simulink library "three_phase_dab_modulator"  (R2025b)
settings: Solver=VariableStepAuto  StartTime=0.0  StopTime=10.0  RelTol=1e-3
undefined symbols (not defined in the file): tc
libraries: SV_pattern_generator_with_global_TRGO x2
settings Model: Creator=dbagn  LastModifiedBy=dbagn

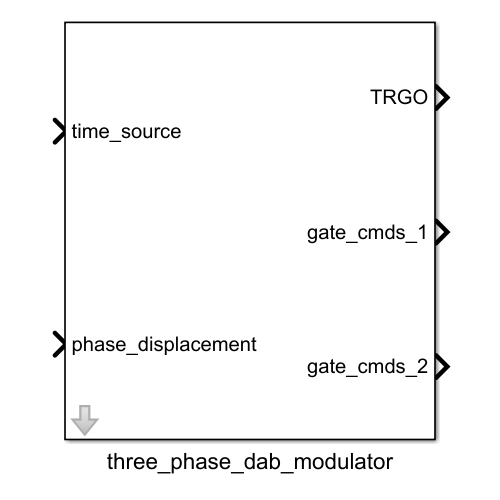
[thumbnail: Simulink's stored preview of the top-level diagram]
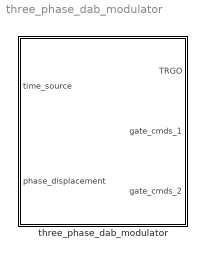
== system three_phase_dab_modulator ==
  three_phase_dab_modulator : Subsystem  mask{fpwm=2400, dead_time=0, tc=tc}
      mask prompts: fpwm "fpwm (Hz)"; dead_time "dead_time (s)"; tc "sampling time (s)"

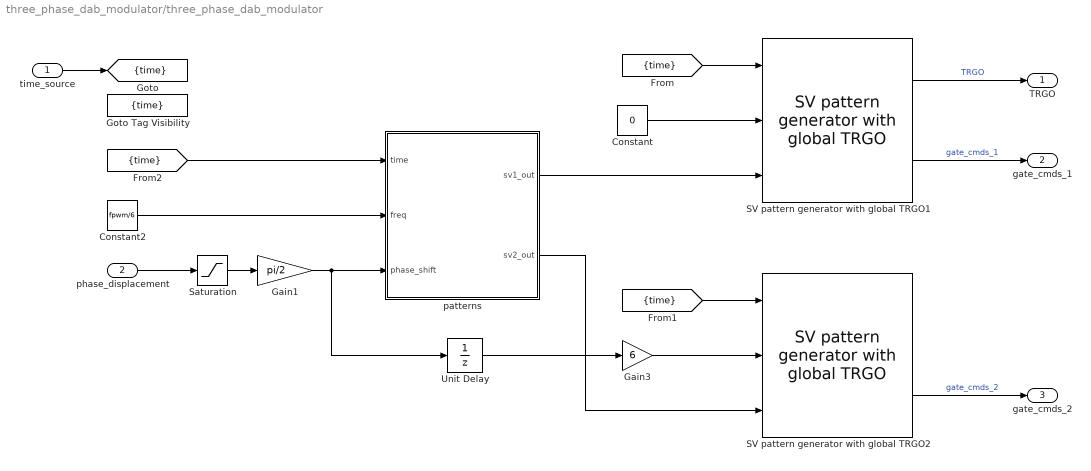
== system three_phase_dab_modulator/three_phase_dab_modulator ==
  time_source : Inport
  phase_displacement : Inport  Port=2
  Constant : Constant  Value=0
  Constant2 : Constant  Value=fpwm/6
  Gain1 : Gain  Gain=pi/2
  Gain3 : Gain  Gain=6
  Goto Tag Visibility : GotoTagVisibility  GotoTag=time
  SV pattern generator with global TRGO1 : SV_pattern_generator_with_global_TRGO/SV pattern generator with global TRGO  f=fpwm  m_up=0.98  m_low=0.02  dead_time=dead_time  pos_cmd_gate=15  neg_cmd_gate=-10  tc=tc
  SV pattern generator with global TRGO2 : SV_pattern_generator_with_global_TRGO/SV pattern generator with global TRGO  f=fpwm  m_up=0.98  m_low=0.02  dead_time=dead_time  pos_cmd_gate=15  neg_cmd_gate=-10  tc=tc
  Saturation : Saturate  UpperLimit=1  LowerLimit=-1
  Unit Delay : UnitDelay  SampleTime=tc  HasFrameUpgradeWarning=on
  patterns : Subsystem
  TRGO : Outport
  gate_cmds_1 : Outport  Port=2
  gate_cmds_2 : Outport  Port=3
  tag scope: time=scoped
  wires:
  SV pattern generator with global TRGO1/2 -> gate_cmds_1/1  "gate_cmds_1"
  Gain3/1 -> SV pattern generator with global TRGO2/2
  Constant/1 -> SV pattern generator with global TRGO1/2
  Constant2/1 -> patterns/2(freq)
  patterns/2(sv2_out) -> SV pattern generator with global TRGO2/3
  patterns/1(sv1_out) -> SV pattern generator with global TRGO1/3
  SV pattern generator with global TRGO1/1 -> TRGO/1  "TRGO"
  phase_displacement/1 -> Saturation/1
  SV pattern generator with global TRGO2/2 -> gate_cmds_2/1  "gate_cmds_2"
  time_source/1 -> [time]
  [time] -> SV pattern generator with global TRGO1/1
  [time] -> SV pattern generator with global TRGO2/1
  [time] -> patterns/1(time)
  Unit Delay/1 -> Gain3/1
  Gain1/1 -> Unit Delay/1, patterns/3(phase_shift)
  Saturation/1 -> Gain1/1

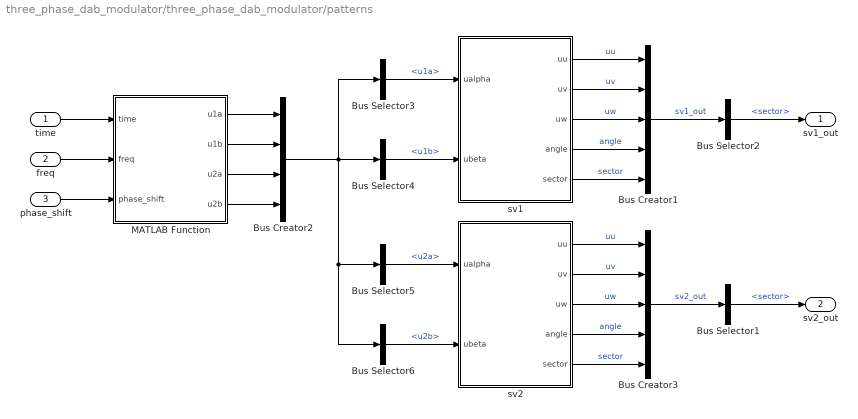
== system three_phase_dab_modulator/three_phase_dab_modulator/patterns ==
  time : Inport
  freq : Inport  Port=2
  phase_shift : Inport  Port=3
  Bus Creator1 : BusCreator  Inputs=5
  Bus Creator2 : BusCreator  Inputs=4
  Bus Creator3 : BusCreator  Inputs=5
  Bus Selector1 : BusSelector  OutputSignals=sector
  Bus Selector2 : BusSelector  OutputSignals=sector
  Bus Selector3 : BusSelector  OutputSignals=u1a
  Bus Selector4 : BusSelector  OutputSignals=u1b
  Bus Selector5 : BusSelector  OutputSignals=u2a
  Bus Selector6 : BusSelector  OutputSignals=u2b
  MATLAB Function : MATLAB Function  TreatAsAtomicUnit=on  SystemSampleTime=tc
  sv1 : MATLAB Function  TreatAsAtomicUnit=on  SystemSampleTime=tc
  sv2 : MATLAB Function  TreatAsAtomicUnit=on  SystemSampleTime=tc
  sv1_out : Outport
  sv2_out : Outport  Port=2
  wires:
  sv2/5(sector) -> Bus Creator3/5  "sector"
  Bus Selector6/1 -> sv2/2(ubeta)  "<u2b>"
  Bus Selector5/1 -> sv2/1(ualpha)  "<u2a>"
  sv2/3(uw) -> Bus Creator3/3  "uw"
  sv1/3(uw) -> Bus Creator1/3  "uw"
  sv2/2(uv) -> Bus Creator3/2  "uv"
  sv2/1(uu) -> Bus Creator3/1  "uu"
  sv2/4(angle) -> Bus Creator3/4  "angle"
  Bus Selector3/1 -> sv1/1(ualpha)  "<u1a>"
  sv1/4(angle) -> Bus Creator1/4  "angle"
  sv1/1(uu) -> Bus Creator1/1  "uu"
  Bus Selector4/1 -> sv1/2(ubeta)  "<u1b>"
  sv1/5(sector) -> Bus Creator1/5  "sector"
  sv1/2(uv) -> Bus Creator1/2  "uv"
  Bus Creator1/1 -> Bus Selector2/1  "sv1_out"
  Bus Selector2/1 -> sv1_out/1  "<sector>"
  Bus Creator3/1 -> Bus Selector1/1  "sv2_out"
  Bus Selector1/1 -> sv2_out/1  "<sector>"
  phase_shift/1 -> MATLAB Function/3(phase_shift)
  time/1 -> MATLAB Function/1(time)
  freq/1 -> MATLAB Function/2(freq)
  MATLAB Function/4(u2b) -> Bus Creator2/4
  MATLAB Function/3(u2a) -> Bus Creator2/3
  MATLAB Function/2(u1b) -> Bus Creator2/2
  MATLAB Function/1(u1a) -> Bus Creator2/1
  Bus Creator2/1 -> Bus Selector3/1, Bus Selector4/1, Bus Selector6/1, Bus Selector5/1

== matlab function three_phase_dab_modulator/patterns/sv1 ==
  data: ualpha input; uu output; ubeta input; uv output; uw output; angle output; sector output
function [uu, uv, uw, angle, sector] = sv(ualpha, ubeta)
% SV: Space Vector duty calculation from Clarke (alpha,beta)
% Inputs: ualpha, ubeta  (assumed normalized to reference)
% Outputs: uu,uv,uw (phase duty ratios 0..1), angle (0..2*pi)

% compute angle in [0,2*pi)
angle = mod(atan2(ubeta, ualpha), 2*pi);

% sector 1..6
sector = floor(angle / (pi/3)) + 1;
if sector > 6, sector = 6; end

% compute t1, t2 for each sector (explicitly)
switch sector
    case 1  % 0 .. pi/3
        t1 =  ualpha - ubeta/sqrt(3);    % v1 contribution
        t2 =  2*ubeta/sqrt(3);           % v2 contribution
    case 2  % pi/3 .. 2*pi/3
        t1 = -ualpha + ubeta/sqrt(3);    % v3
        t2 =  ualpha + ubeta/sqrt(3);    % v2
    case 3  % 2*pi/3 .. pi
        t1 =  2*ubeta/sqrt(3);           % v3
        t2 = -ualpha - ubeta/sqrt(3);    % v4
    case 4  % pi .. 4*pi/3
        t1 = -2*ubeta/sqrt(3);           % v5
        t2 =  ubeta/sqrt(3) - ualpha;    % v4
    case 5  % 4*pi/3 .. 5*pi/3
        t1 = -ualpha - ubeta/sqrt(3);    % v5
        t2 =  ualpha - ubeta/sqrt(3);    % v6
    case 6  % 5*pi/3 .. 2*pi
        t1 =  ualpha + ubeta/sqrt(3);    % v1
        t2 = -2*ubeta/sqrt(3);           % v6
    otherwise
        t1 = 0; t2 = 0;
end

% safety: ensure t1,t2 are non-negative in pathological inputs
% (these expressions can be negative depending on ualpha/ubeta signs;
%  we rely on sector selection to produce correct relative signs, but
%  still protect t0 below)
% compute t0
t0 = 1 - (t1 + t2);

% if t0 is negative, scale t1,t2 so that t0 = 0 (avoid negative dwell)
if t0 < 0
    s = 1 / (t1 + t2);    % scale to make t1+t2 == 1
    t1 = t1 * s;
    t2 = t2 * s;
    t0 = 0;
end

% compute phase duty values according to sector mapping
switch sector
    case 1
        ua = t0/2;
        ub = ua + t1;
        uc = ub + t2;
    case 2
        ub = t0/2;
        ua = ub + t1;
        uc = ua + t2;
    case 3
        ub = t0/2;
        uc = ub + t1;
        ua = uc + t2;
    case 4
        uc = t0/2;
        ub = uc + t1;
        ua = ub + t2;
    case 5
        uc = t0/2;
        ua = uc + t1;
        ub = ua + t2;
    case 6
        ua = t0/2;
        uc = ua + t1;
        ub = uc + t2;
    otherwise
        ua = 0; ub = 0; uc = 0;
end

% output
uu = ua;
uv = ub;
uw = uc;
end

== matlab function three_phase_dab_modulator/patterns/sv2 ==
  data: ualpha input; uu output; ubeta input; uv output; uw output; angle output; sector output
function [uu, uv, uw, angle, sector] = sv(ualpha, ubeta)
% SV: Space Vector duty calculation from Clarke (alpha,beta)
% Inputs: ualpha, ubeta  (assumed normalized to reference)
% Outputs: uu,uv,uw (phase duty ratios 0..1), angle (0..2*pi)

% compute angle in [0,2*pi)
angle = mod(atan2(ubeta, ualpha), 2*pi);

% sector 1..6
sector = floor(angle / (pi/3)) + 1;
if sector > 6, sector = 6; end

% compute t1, t2 for each sector (explicitly)
switch sector
    case 1  % 0 .. pi/3
        t1 =  ualpha - ubeta/sqrt(3);    % v1 contribution
        t2 =  2*ubeta/sqrt(3);           % v2 contribution
    case 2  % pi/3 .. 2*pi/3
        t1 = -ualpha + ubeta/sqrt(3);    % v3
        t2 =  ualpha + ubeta/sqrt(3);    % v2
    case 3  % 2*pi/3 .. pi
        t1 =  2*ubeta/sqrt(3);           % v3
        t2 = -ualpha - ubeta/sqrt(3);    % v4
    case 4  % pi .. 4*pi/3
        t1 = -2*ubeta/sqrt(3);           % v5
        t2 =  ubeta/sqrt(3) - ualpha;    % v4
    case 5  % 4*pi/3 .. 5*pi/3
        t1 = -ualpha - ubeta/sqrt(3);    % v5
        t2 =  ualpha - ubeta/sqrt(3);    % v6
    case 6  % 5*pi/3 .. 2*pi
        t1 =  ualpha + ubeta/sqrt(3);    % v1
        t2 = -2*ubeta/sqrt(3);           % v6
    otherwise
        t1 = 0; t2 = 0;
end

% safety: ensure t1,t2 are non-negative in pathological inputs
% (these expressions can be negative depending on ualpha/ubeta signs;
%  we rely on sector selection to produce correct relative signs, but
%  still protect t0 below)
% compute t0
t0 = 1 - (t1 + t2);

% if t0 is negative, scale t1,t2 so that t0 = 0 (avoid negative dwell)
if t0 < 0
    s = 1 / (t1 + t2);    % scale to make t1+t2 == 1
    t1 = t1 * s;
    t2 = t2 * s;
    t0 = 0;
end

% compute phase duty values according to sector mapping
switch sector
    case 1
        ua = t0/2;
        ub = ua + t1;
        uc = ub + t2;
    case 2
        ub = t0/2;
        ua = ub + t1;
        uc = ua + t2;
    case 3
        ub = t0/2;
        uc = ub + t1;
        ua = uc + t2;
    case 4
        uc = t0/2;
        ub = uc + t1;
        ua = ub + t2;
    case 5
        uc = t0/2;
        ua = uc + t1;
        ub = ua + t2;
    case 6
        ua = t0/2;
        uc = ua + t1;
        ub = uc + t2;
    otherwise
        ua = 0; ub = 0; uc = 0;
end

% output
uu = ua;
uv = ub;
uw = uc;
end

== matlab function three_phase_dab_modulator/patterns/MATLAB Function ==
  data: time input; u1a output; freq input; phase_shift input; u1b output; u2a output; u2b output
function [u1a,u1b,u2a,u2b] = fcn(time, freq, phase_shift)

u1a = cos(2*pi*freq*time -pi/2);
u1b = sin(2*pi*freq*time -pi/2);
u2a = cos(2*pi*freq*time -pi/2 - phase_shift);
u2b = sin(2*pi*freq*time -pi/2 - phase_shift);
